simulink model "Regulator2"  (R2023b)
settings: Solver=FixedStepAuto  StartTime=0.0  StopTime=40  FixedStep=0.001  RelTol=1e-3
values from neighbouring files (symbols this model uses):
  B_e = 0.05    [GA.m]    (also in exam.m = 0.001; grafs.m = gears(i); pi_GA.m; test.m = 0.001)
  B_m = 0.000080292    (= 8.0292e-05)    [GA.m]    (also in exam.m; pi_GA.m; test.m)
  B_z = 0.00020000    (= 0.0002)    [GA.m]    (also in exam.m; pi_GA.m; test.m)
  i = 5    [exam.m]
  J_m = 0.00009    (= 9e-05)    [GA.m]    (also in exam.m; pi_GA.m; test.m)
  J_z = 0.00024943    [GA.m]    (also in exam.m; pi_GA.m; test.m)
  K_e = 0.5    [GA.m]    (also in exam.m = 0.01; grafs.m = gears(i); pi_GA.m; test.m = 0.01)
  M_m = 0.108    [GA.m]    (also in exam.m; pi_GA.m; test.m)
  M_z0m = 0.0052    [GA.m]    (also in exam.m; pi_GA.m; test.m)
  M_z0z = 0.0078    [GA.m]    (also in exam.m; pi_GA.m; test.m)
  N_el = 10000    [GA.m]    (also in exam.m; pi_GA.m; test.m)
  T_n = 0.001    [GA.m]    (also in exam.m; pi_GA.m; test.m)
  T_vz = 0.001    [GA.m]    (also in exam.m; pi_GA.m; test.m)
undefined symbols (not defined in the file or in its folder): DiscIntNeverNeededParam, param
settings Model: Creator=timip  LastModifiedBy=maros-pc
settings SolverCC: ConsecutiveZCsStepRelTol=1000*128*eps  ZeroCrossAlgorithm=Adaptive  EnableFixedStepZeroCrossing=on  MaxZcPerStep=5

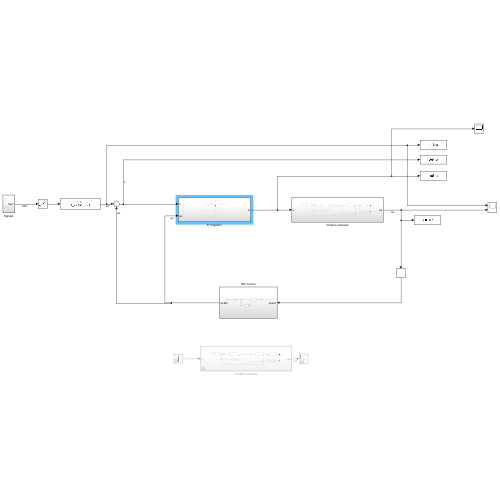
[thumbnail: Simulink's stored preview of the top-level diagram]
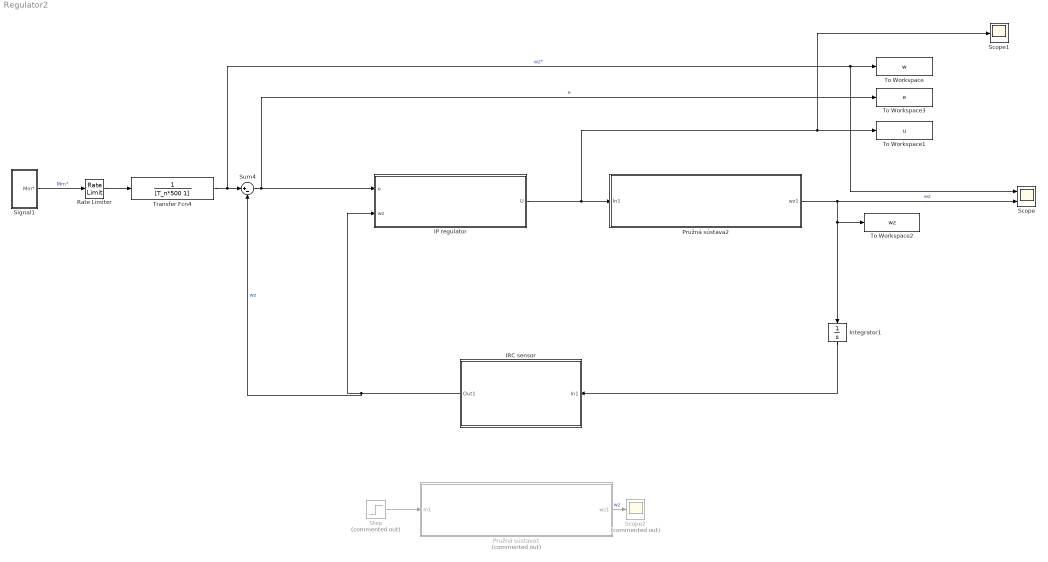
== system Regulator2 ==
  IP regulator : Subsystem
  IRC sensor : Subsystem
  Integrator1 : Integrator
  Pružná sústava1 : Subsystem  Commented=on
  Pružná sústava2 : Subsystem
  Rate Limiter : RateLimiter  RisingSlewLimit=0.8  FallingSlewLimit=-0.8  SampleTimeMode=inherited
  Scope : Scope  NumInputPorts=2
  Scope1 : Scope
  Scope2 : Scope  Commented=on
  Signal1 : Subsystem
  Step : Step  Commented=on  SampleTime=0
  Sum4 : Sum  Inputs=|+-
  To Workspace : ToWorkspace  VariableName=w  SaveFormat=Timeseries  SampleTime=-1
  To Workspace1 : ToWorkspace  VariableName=u  SaveFormat=Timeseries  SampleTime=-1
  To Workspace2 : ToWorkspace  VariableName=wz  SaveFormat=Timeseries  SampleTime=-1
  To Workspace3 : ToWorkspace  VariableName=e  SaveFormat=Timeseries  SampleTime=-1
  Transfer Fcn4 : TransferFcn  Denominator=[T_n*500 1]
  wires:
  Sum4/1 -> To Workspace3/1, IP regulator/1(e)  "e"
  Transfer Fcn4/1 -> Sum4/1, Scope/1, To Workspace/1  "wz*"
  Rate Limiter/1 -> Transfer Fcn4/1
  Integrator1/1 -> IRC sensor/1(In1)
  IRC sensor/1(Out1) -> Sum4/2, IP regulator/2(wz)  "wz"
  IP regulator/1(U) -> Pružná sústava2/1(In1), Scope1/1, To Workspace1/1
  Pružná sústava2/1(wz1) -> To Workspace2/1, Integrator1/1, Scope/2  "wz"
  Signal1/1(Mm*) -> Rate Limiter/1  "Mm*"
  Pružná sústava1/1(wz1) -> Scope2/1  "wz"
  Step/1 -> Pružná sústava1/1(In1)

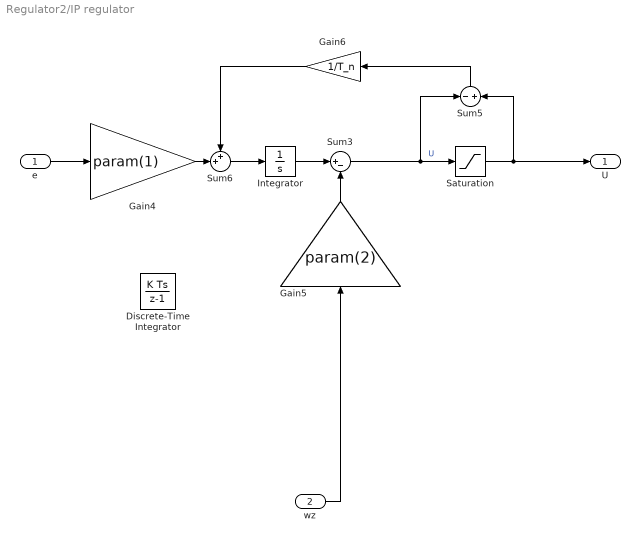
== system Regulator2/IP regulator ==
  e : Inport
  wz : Inport  Port=2
  Discrete-Time Integrator : DiscreteIntegrator  SampleTime=-1  ICPrevOutput=DiscIntNeverNeededParam  ICPrevScaledInput=DiscIntNeverNeededParam
  Gain4 : Gain  Gain=param(1)
  Gain5 : Gain  Gain=param(2)
  Gain6 : Gain  Gain=1/T_n
  Integrator : Integrator
  Saturation : Saturate  UpperLimit=M_m*0.75  LowerLimit=-M_m*0.75
  Sum3 : Sum  Inputs=|+-
  Sum5 : Sum  Inputs=-+
  Sum6 : Sum  Inputs=++|
  U : Outport
  wires:
  Gain5/1 -> Sum3/2
  Gain4/1 -> Sum6/2
  Saturation/1 -> U/1, Sum5/2  "U"
  Sum5/1 -> Gain6/1
  Integrator/1 -> Sum3/1
  Gain6/1 -> Sum6/1
  Sum3/1 -> Sum5/1, Saturation/1
  Sum6/1 -> Integrator/1
  wz/1 -> Gain5/1
  e/1 -> Gain4/1

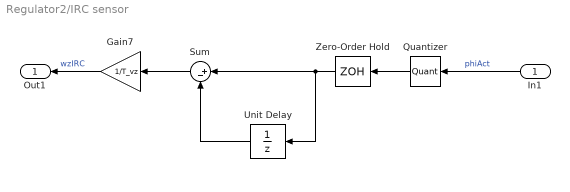
== system Regulator2/IRC sensor ==
  In1 : Inport
  Gain7 : Gain  Gain=1/T_vz
  Quantizer : Quantizer  QuantizationInterval=2*pi/N_el
  Sum : Sum  Inputs=|+-
  Unit Delay : UnitDelay  SampleTime=-1  HasFrameUpgradeWarning=on
  Zero-Order Hold : ZeroOrderHold  SampleTime=T_vz
  Out1 : Outport
  wires:
  Unit Delay/1 -> Sum/2
  Quantizer/1 -> Zero-Order Hold/1
  Zero-Order Hold/1 -> Unit Delay/1, Sum/1
  Gain7/1 -> Out1/1  "wzIRC"
  In1/1 -> Quantizer/1  "phiAct"
  Sum/1 -> Gain7/1

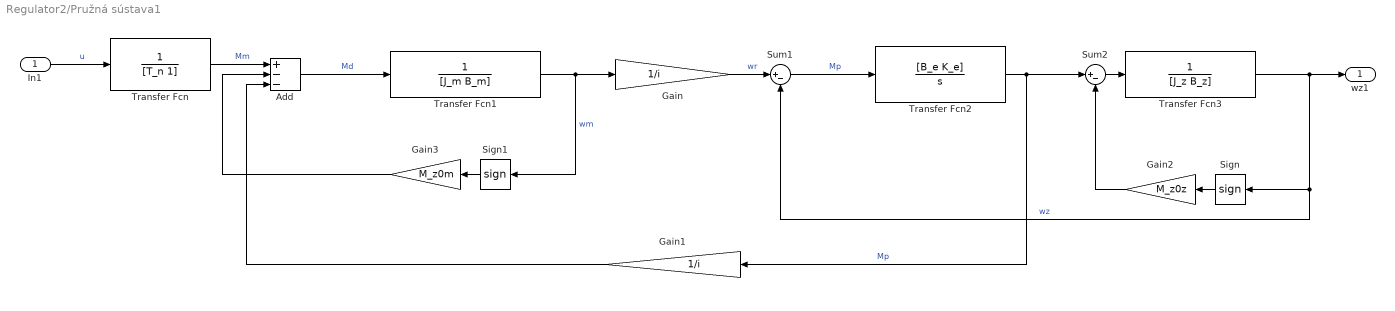
== system Regulator2/Pružná sústava1 ==
  In1 : Inport
  Add : Sum  Inputs=+--
  Gain : Gain  Gain=1/i
  Gain1 : Gain  Gain=1/i
  Gain2 : Gain  Gain=M_z0z
  Gain3 : Gain  Gain=M_z0m
  Sign : Signum
  Sign1 : Signum
  Sum1 : Sum  Inputs=|+-
  Sum2 : Sum  Inputs=|+-
  Transfer Fcn : TransferFcn  Denominator=[T_n 1]
  Transfer Fcn1 : TransferFcn  Denominator=[J_m B_m]
  Transfer Fcn2 : TransferFcn  Numerator=[B_e K_e]  Denominator=[1 0]
  Transfer Fcn3 : TransferFcn  Denominator=[J_z B_z]
  wz1 : Outport
  wires:
  Transfer Fcn/1 -> Add/1  "Mm"
  Transfer Fcn1/1 -> Sign1/1, Gain/1  "wm"
  Sign/1 -> Gain2/1
  Gain/1 -> Sum1/1  "wr"
  Gain1/1 -> Add/3
  In1/1 -> Transfer Fcn/1  "u"
  Sign1/1 -> Gain3/1
  Sum2/1 -> Transfer Fcn3/1
  Sum1/1 -> Transfer Fcn2/1  "Mp"
  Transfer Fcn2/1 -> Gain1/1, Sum2/1  "Mp"
  Gain3/1 -> Add/2
  Add/1 -> Transfer Fcn1/1  "Md"
  Gain2/1 -> Sum2/2
  Transfer Fcn3/1 -> Sign/1, Sum1/2, wz1/1  "wz"

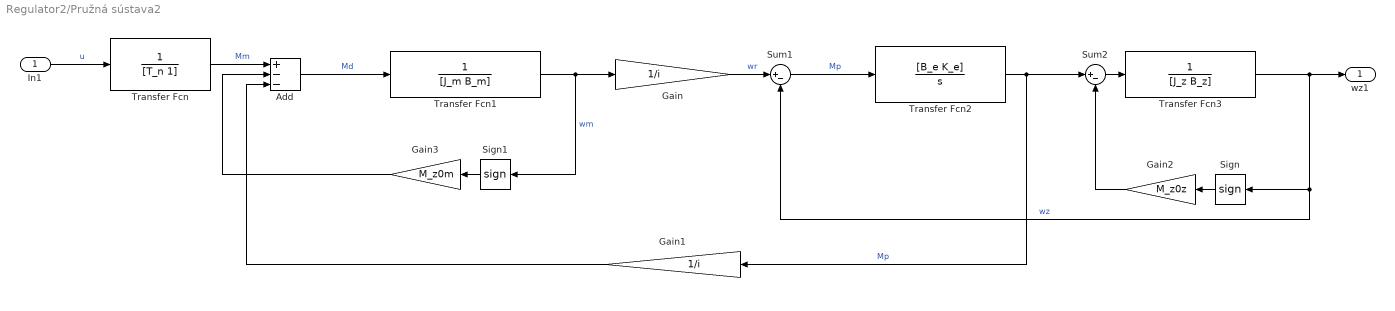
== system Regulator2/Pružná sústava2 ==
  In1 : Inport
  Add : Sum  Inputs=+--
  Gain : Gain  Gain=1/i
  Gain1 : Gain  Gain=1/i
  Gain2 : Gain  Gain=M_z0z
  Gain3 : Gain  Gain=M_z0m
  Sign : Signum
  Sign1 : Signum
  Sum1 : Sum  Inputs=|+-
  Sum2 : Sum  Inputs=|+-
  Transfer Fcn : TransferFcn  Denominator=[T_n 1]
  Transfer Fcn1 : TransferFcn  Denominator=[J_m B_m]
  Transfer Fcn2 : TransferFcn  Numerator=[B_e K_e]  Denominator=[1 0]
  Transfer Fcn3 : TransferFcn  Denominator=[J_z B_z]
  wz1 : Outport
  wires:
  Transfer Fcn/1 -> Add/1  "Mm"
  Transfer Fcn1/1 -> Sign1/1, Gain/1  "wm"
  Sign/1 -> Gain2/1
  Gain/1 -> Sum1/1  "wr"
  Gain1/1 -> Add/3
  In1/1 -> Transfer Fcn/1  "u"
  Sign1/1 -> Gain3/1
  Sum2/1 -> Transfer Fcn3/1
  Sum1/1 -> Transfer Fcn2/1  "Mp"
  Transfer Fcn2/1 -> Gain1/1, Sum2/1  "Mp"
  Gain3/1 -> Add/2
  Add/1 -> Transfer Fcn1/1  "Md"
  Gain2/1 -> Sum2/2
  Transfer Fcn3/1 -> Sign/1, Sum1/2, wz1/1  "wz"

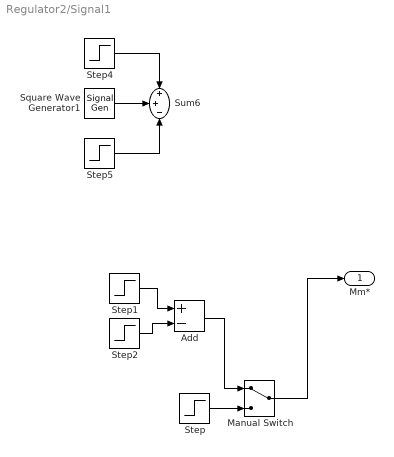
== system Regulator2/Signal1 ==
  Add : Sum  Inputs=+-
  Manual Switch : ManualSwitch
  Square Wave Generator1 : SignalGenerator  Amplitude=0.8  Frequency=2
  Step : Step  SampleTime=0
  Step1 : Step  After=pi  SampleTime=0
  Step2 : Step  Time=10  After=pi  SampleTime=0
  Step4 : Step  SampleTime=0
  Step5 : Step  Time=2  SampleTime=0
  Sum6 : Sum  Inputs=++-
  Mm* : Outport
  wires:
  Step4/1 -> Sum6/1
  Manual Switch/1 -> Mm*/1
  Square Wave Generator1/1 -> Sum6/2
  Step5/1 -> Sum6/3
  Step/1 -> Manual Switch/2
  Add/1 -> Manual Switch/1
  Step1/1 -> Add/1
  Step2/1 -> Add/2
